simulink model "test_sys_MHE"  (R2022b)
settings: Solver=FixedStepDiscrete  StartTime=0.0  StopTime=T_final  FixedStep=T_sample  RelTol=1e-3
values from neighbouring files (symbols this model uses):
  A = [0.4 -0.3 0 0.1 ... (first row only)    [Q1_experiment.m]    (also in Run_model.m = [0.921 0 0.041 0; To_Tobias.m = [0.921 0 0.041 0; test.m)
  A_ineq = -[zeros(1,n_alpha) zeros(1,n_states*L) zeros(1,n_meas*L) ... (first row only)    [Run_model.m]
  Aeq = [HL_u zeros(size(HL_u,1),n_states*L) zeros(size(HL_u,1),n_meas*L) ... (first row only)    [Run_model.m]
  B = [0; -1; 1.4; 0]    [Q1_experiment.m]    (also in Run_model.m = [0.017 0.001; To_Tobias.m = [0.017 0.001; test.m)
  b_ineq = zeros(1+n_states*L+n_meas*L,1)    [Run_model.m]
  C = [-0.7 0 -2 0.4]    [Q1_experiment.m]    (also in Run_model.m = [1 0 0 0; To_Tobias.m = [1 0 0 0; test.m = [-0.7 0 -2 0.4)
  D = 0.2    [Q1_experiment.m]    (also in Run_model.m = zeros(n_meas,n_int); To_Tobias.m = zeros(n_meas,n_int); test.m)
  f = [zeros(1,n_states) ... (first row only)    [Run_model.m]
  H = zeros(m*L,N-L+1)    [Get_Hankel.m]    (also in Get_Hankel_adj.m = kron(H_alph,eye(n)); Run_model.m = [H1)
  L = 5    [Q1_experiment.m]    (also in Run_model.m = 7; To_Tobias.m; test.m = 2)
  n_states = size(A,1)    [test.m]
  T_start_opt = T_sample*(L+1)    (= 0.08)    [Run_model.m]    (also in To_Tobias.m = 0.06)
  U0 = zeros(n_int,L+1)    [Run_model.m]    (also in To_Tobias.m)
  x0 = zeros(n_states,1)    [Q1_experiment.m]    (also in Run_model.m = 7*ones(n_states,1); To_Tobias.m = 7*ones(n_states,1); test.m = rand(n_states,1))
  X0_hat = kron(ones(L,1),x0_hat)    [Run_model.m]    (also in To_Tobias.m)
  Y0 = zeros(n_meas,L)    [Run_model.m]    (also in To_Tobias.m)
libraries: simulink x1
settings Model: Creator=Abelb  LastModifiedBy=RASLab-Distributed
settings DebuggingCC: UnconnectedInputMsg=warning  UnconnectedOutputMsg=warning  UnconnectedLineMsg=warning
settings ModelReferenceCC: EnableRefExpFcnMdlSchedulingChecks=on
settings RTWCC: DLArmComputeVersion=19.05

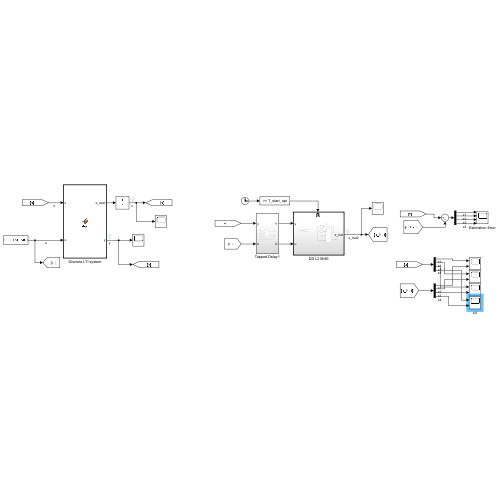
[thumbnail: Simulink's stored preview of the top-level diagram]
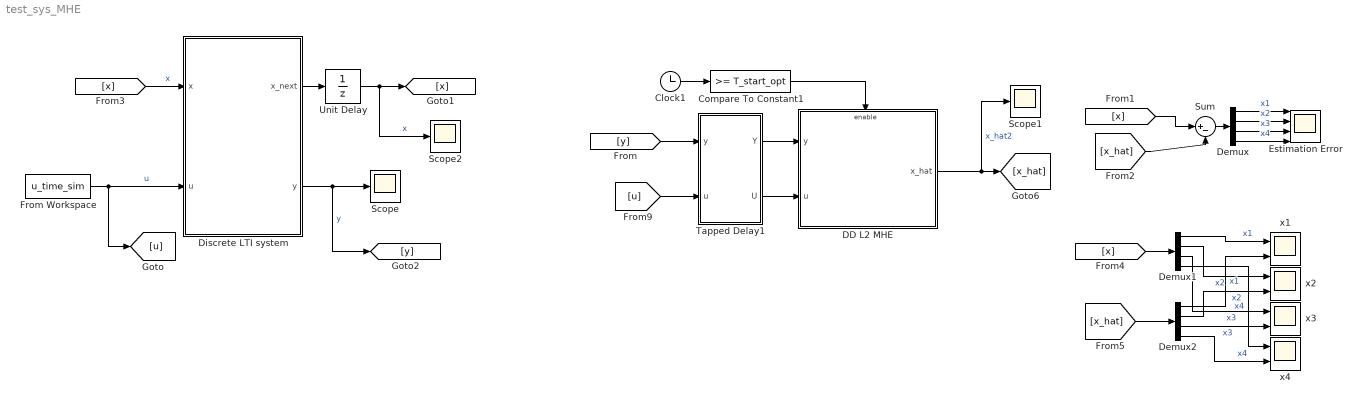
== system test_sys_MHE ==
  Clock1 : Clock
  Compare To Constant1 : simulink/Logic and Bit Operations/Compare To Constant  relop=>=  const=T_start_opt  OutDataTypeStr=boolean
  DD L2 MHE : Subsystem
  Demux : Demux
  Demux1 : Demux
  Demux2 : Demux
  Discrete LTI system : MATLAB Function  TreatAsAtomicUnit=on
  Estimation Error : Scope  NumInputPorts=4
  From Workspace : FromWorkspace  VariableName=u_time_sim
  Scope : Scope
  Scope1 : Scope
  Scope2 : Scope
  Sum : Sum  Inputs=|+-
  Tapped Delay1 : Subsystem
  Unit Delay : UnitDelay  InitialCondition=x0  SampleTime=-1  HasFrameUpgradeWarning=on
  x{1..4} (4 alike) : Scope  NumInputPorts=2
  wires:
  Discrete LTI system/1(x_next) -> Unit Delay/1
  From Workspace/1 -> [u], Discrete LTI system/2(u)  "u"
  Unit Delay/1 -> Scope2/1, [x]  "x"
  [x] -> Discrete LTI system/1(x)  "x"
  Discrete LTI system/2(y) -> [y], Scope/1  "y"
  Tapped Delay1/2(U) -> DD L2 MHE/2(u)
  Tapped Delay1/1(Y) -> DD L2 MHE/1(y)
  DD L2 MHE/1(x_hat) -> Scope1/1, [x_hat]  "x_hat2"
  [u] -> Tapped Delay1/2(u)
  [y] -> Tapped Delay1/1(y)
  Clock1/1 -> Compare To Constant1/1
  Compare To Constant1/1 -> DD L2 MHE/Enable
  [x_hat] -> Sum/2
  [x] -> Sum/1
  Sum/1 -> Demux/1
  Demux/1 -> Estimation Error/1  "x1"
  Demux/2 -> Estimation Error/2  "x2"
  Demux/3 -> Estimation Error/3  "x3"
  Demux/4 -> Estimation Error/4  "x4"
  [x] -> Demux1/1
  [x_hat] -> Demux2/1
  Demux1/1 -> x1/1  "x1"
  Demux2/1 -> x1/2  "x1"
  Demux1/2 -> x2/1  "x2"
  Demux2/2 -> x2/2  "x2"
  Demux1/3 -> x3/1  "x3"
  Demux2/3 -> x3/2  "x3"
  Demux1/4 -> x4/1  "x4"
  Demux2/4 -> x4/2  "x4"

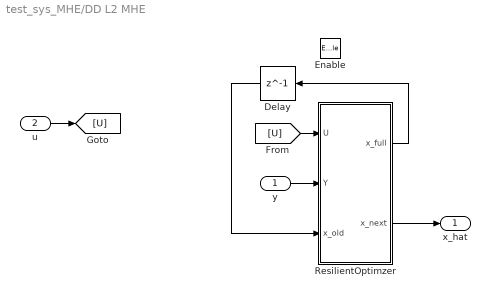
== system test_sys_MHE/DD L2 MHE ==
  y : Inport
  u : Inport  Port=2
  Enable : EnablePort
  Delay : Delay  DelayLength=1  InitialCondition=X0_hat
  ResilientOptimzer : MATLAB Function  TreatAsAtomicUnit=on
  x_hat : Outport
  wires:
  u/1 -> [U]
  y/1 -> ResilientOptimzer/2(Y)
  [U] -> ResilientOptimzer/1(U)
  ResilientOptimzer/2(x_next) -> x_hat/1
  ResilientOptimzer/1(x_full) -> Delay/1
  Delay/1 -> ResilientOptimzer/3(x_old)

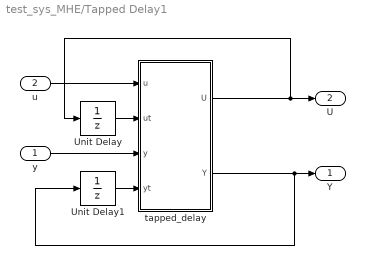
== system test_sys_MHE/Tapped Delay1 ==
  y : Inport
  u : Inport  Port=2
  Unit Delay : UnitDelay  InitialCondition=U0  SampleTime=-1  HasFrameUpgradeWarning=on
  Unit Delay1 : UnitDelay  InitialCondition=Y0  SampleTime=-1  HasFrameUpgradeWarning=on
  tapped_delay : MATLAB Function  TreatAsAtomicUnit=on
  Y : Outport
  U : Outport  Port=2
  wires:
  u/1 -> tapped_delay/1(u)
  y/1 -> tapped_delay/3(y)
  tapped_delay/1(U) -> Unit Delay/1, U/1
  tapped_delay/2(Y) -> Unit Delay1/1, Y/1
  Unit Delay/1 -> tapped_delay/2(ut)
  Unit Delay1/1 -> tapped_delay/4(yt)

== matlab function test_sys_MHE/DD L2 MHE/ResilientOptimzer ==
  data: x_full output; x_next output; U input; Y input; x_old input; H parameter; n_states parameter; L parameter; f parameter; Aeq parameter; A_ineq parameter; b_ineq parameter
function [x_full,x_next]   = fcn(U,Y,x_old,H,n_states,L, f, Aeq,A_ineq, b_ineq)          
%% DD L2
%% function [x_next,r]  = fcn(U,Y, Aeq,n_states,E_MH,T, DE_MH, n_alpha, CE_MH)

% vectorized
u_local = U(:,2:end);
u = u_local(:);
y = Y(:);

% x_old_hat = x_old(n_states+1:2*n_states,:);
beq = [u;y;zeros(n_states*L,1)];
% 
% z_hat = quadprog(H.'*H,x_old_hat.'*f.'*H,[],[],Aeq,beq);
% 
% x_full = z_hat(end-n_states*L+1:end,:);
coder.extrinsic('mhe');

x_full = zeros(n_states*L,1);
x_full(:) = mhe(x_old,beq,Aeq,A_ineq,b_ineq,H,f,n_states,L);
x_next = x_full(1:n_states,:);

== matlab function test_sys_MHE/Tapped Delay1/tapped_delay ==
  data: u input; U output; ut input; y input; yt input; Y output
function [U,Y] = fcn(u,ut,y,yt)
%% tapped_delay_array
% shift columns from tapped matrix to the left and appends most recent
% vector to the last column
%%% input
ut(:,1:end-1) = ut(:,2:end);
ut(:,end) = u;
U = ut;
%%% output
yt(:,1:end-1) = yt(:,2:end);
yt(:,end) = y;
Y = yt;

== matlab function test_sys_MHE/Discrete LTI system ==
  data: x input; x_next output; u input; y output; A parameter; C parameter; B parameter; D parameter
function [x_next,y] = fcn(x,u,A,C,B,D)
% Discrete state-space model for system

x_next = A*x + B*u;

y = C*x + D*u;
